simulink model "test2"  (Simulink 7.5)
settings: Solver=ode15s  StartTime=0.0  StopTime=50  RelTol=1e-3
libraries: powerlib x16, powerlib_extras x2
settings Model: Creator=lm  LastModifiedBy=lm

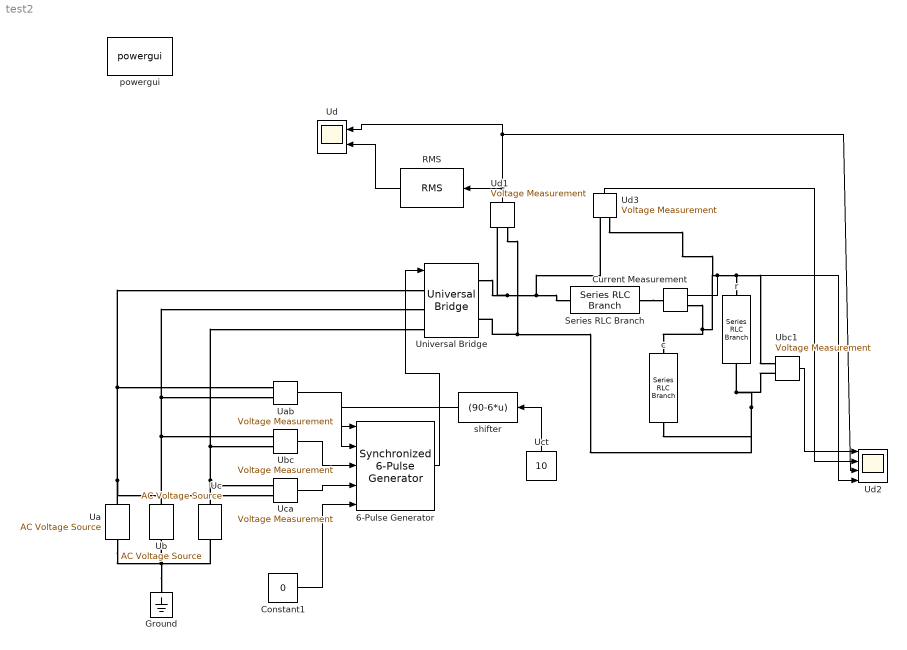
== system test2 ==
  6-Pulse Generator : powerlib_extras/Control  Blocks/Synchronized 6-Pulse Generator  DialogController=POWERSYS.PowerSysDialog  SystemSampleTime=-1  freq=50  pwidth=5  Double_Pulse=on
  Constant1 : Constant  Value=0  OutDataType=fixdt(1, 16)  OutScaling=2^0
  Current Measurement : powerlib/Measurements/Current Measurement  DialogController=POWERSYS.PowerSysDialog  SystemSampleTime=-1  PhasorSimulation=off  OutputType=Complex  PSBequivalent=0
  Ground : powerlib/Elements/Ground  DialogController=POWERSYS.PowerSysDialog  PhysicalDomain=powersysdomain  SubClassName=unknown  LeftPortType=p1  RightPortType=p1  LConnTagsString=a
  RMS : powerlib_extras/Measurements/RMS  DialogController=POWERSYS.PowerSysDialog  SystemSampleTime=-1  f1=60
  Series RLC Branch : powerlib/Elements/Series RLC Branch  DialogController=POWERSYS.PowerSysDialog  PhysicalDomain=powersysdomain  SubClassName=unknown  LeftPortType=p1  RightPortType=p1  LConnTagsString=__new0  RConnTagsString=__new0  BranchType=RL  Resistance=0.2  Inductance=0.2  SetiL0=off  InitialCurrent=0  Capacitance=1e-6  Setx0=off  InitialVoltage=0  Measurements=None
  Ua : powerlib/Electrical Sources/AC Voltage Source  DialogController=POWERSYS.PowerSysDialog  SystemSampleTime=-1  Amplitude=220*sqrt(2)  Phase=0  Frequency=50  SampleTime=0  Measurements=None
  Uab : powerlib/Measurements/Voltage Measurement  DialogController=POWERSYS.PowerSysDialog  SystemSampleTime=-1  PhasorSimulation=off  OutputType=Complex  PSBequivalent=0
  Ub : powerlib/Electrical Sources/AC Voltage Source  DialogController=POWERSYS.PowerSysDialog  SystemSampleTime=-1  Amplitude=220*sqrt(2)  Phase=-120  Frequency=50  SampleTime=0  Measurements=None
  Ubc : powerlib/Measurements/Voltage Measurement  DialogController=POWERSYS.PowerSysDialog  SystemSampleTime=-1  PhasorSimulation=off  OutputType=Complex  PSBequivalent=0
  Ubc1 : powerlib/Measurements/Voltage Measurement  DialogController=POWERSYS.PowerSysDialog  SystemSampleTime=-1  PhasorSimulation=off  OutputType=Complex  PSBequivalent=0
  Uc : powerlib/Electrical Sources/AC Voltage Source  DialogController=POWERSYS.PowerSysDialog  SystemSampleTime=-1  Amplitude=220*sqrt(2)  Phase=-240  Frequency=50  SampleTime=0  Measurements=None
  Uca : powerlib/Measurements/Voltage Measurement  DialogController=POWERSYS.PowerSysDialog  SystemSampleTime=-1  PhasorSimulation=off  OutputType=Complex  PSBequivalent=0
  Uct : Constant  Value=10  OutDataType=fixdt(1, 16)  OutScaling=2^0
  Ud : Scope  NumInputPorts=2
      settings: YMin=-80~1.7e-005  YMax=0~2.125e-005
  Ud1 : powerlib/Measurements/Voltage Measurement  DialogController=POWERSYS.PowerSysDialog  SystemSampleTime=-1  PhasorSimulation=off  OutputType=Complex  PSBequivalent=0
  Ud2 : Scope  NumInputPorts=4
      settings: TimeRange=4  YMin=362~-125~250~361.5  YMax=362.3~175~550~362.6
  Ud3 : powerlib/Measurements/Voltage Measurement  DialogController=POWERSYS.PowerSysDialog  SystemSampleTime=-1  PhasorSimulation=off  OutputType=Complex  PSBequivalent=0
  Universal Bridge : powerlib/Power Electronics/Universal Bridge  DialogController=POWERSYS.PowerSysDialog  SystemSampleTime=-1  Arms=3  SnubberResistance=1e6  SnubberCapacitance=inf  Device=Thyristors  Ron=0.006  Lon=0  ForwardVoltages="[  0  0  ]"  ForwardVoltage=0  GTOparameters=[ 10e-6 , 20e-6 ]  IGBTparameters=[ 1e-6 , 2e-6 ]  Measurements=Device voltages  Measurements_2=None  converterType=Rectifier
  c : powerlib/Elements/Series RLC Branch  DialogController=POWERSYS.PowerSysDialog  PhysicalDomain=powersysdomain  SubClassName=unknown  LeftPortType=p1  RightPortType=p1  LConnTagsString=__new0  RConnTagsString=__new0  BranchType=C  Resistance=1  Inductance=1e-3  SetiL0=off  InitialCurrent=0  Capacitance=0.1  Setx0=off  InitialVoltage=0  Measurements=None
  powergui : powerlib/powergui  Priority=1  SystemSampleTime=-1  SimulationMode=Discrete  SampleTime=50e-6  frequency=60  SPID=off  DisableSnubberDevices=off  DisableRonSwitches=off  DisableVfSwitches=off  SwTol=0  Interpol=off  frequencyindice=0  echomessages=off  HookPort=off  DisplayEquations=off  FunctionMessages=off  EnableUseOfTLC=off  x0status=blocks  RestoreLinks=warning  ResistiveCurrentMeasurement=off  Ylog=off  Xlog=on  ShowGrid=off  save=off  variable=ZData  ZoomFFT=off  StartTime=0.0  cycles=1  DisplayStyle=1  FreqAxis=off  MaxFrequency=1000  frequencyindicesteady=1  display=off  methode=off
  r : powerlib/Elements/Series RLC Branch  DialogController=POWERSYS.PowerSysDialog  PhysicalDomain=powersysdomain  SubClassName=unknown  LeftPortType=p1  RightPortType=p1  LConnTagsString=__new0  RConnTagsString=__new0  BranchType=R  Resistance=1  Inductance=1e-3  SetiL0=off  InitialCurrent=0  Capacitance=1e-6  Setx0=off  InitialVoltage=0  Measurements=None
  shifter : Fcn  Expr=(90-6*u)
  wires:
  Constant1/1 -> 6-Pulse Generator/5
  Uca/1 -> 6-Pulse Generator/4
  Ubc/1 -> 6-Pulse Generator/3
  Uab/1 -> 6-Pulse Generator/2
  Uct/1 -> shifter/1
  shifter/1 -> 6-Pulse Generator/1
  Ud1/1 -> RMS/1, Ud/1, Ud2/3
  RMS/1 -> Ud/2
  6-Pulse Generator/1 -> Universal Bridge/1
  Ubc1/1 -> Ud2/1
  Ud3/1 -> Ud2/2
  Current Measurement/1 -> Ud2/4
  connections:
  Ground/LConn1 -- Ua/LConn1 -- Ub/LConn1 -- Uc/LConn1
  Ua/RConn1 -- Universal Bridge/LConn1 -- Uab/LConn1 -- Uca/LConn2
  Ub/RConn1 -- Universal Bridge/LConn2 -- Uab/LConn2 -- Ubc/LConn1
  Uc/RConn1 -- Universal Bridge/LConn3 -- Ubc/LConn2 -- Uca/LConn1
  Ud3/LConn1 -- Universal Bridge/RConn1 -- Ud1/LConn1 -- Series RLC Branch/LConn1
  Ud1/LConn2 -- Universal Bridge/RConn2 -- Ubc1/LConn2 -- r/LConn1 -- c/RConn1
  Ud3/LConn2 -- r/RConn1 -- Ubc1/LConn1 -- Current Measurement/RConn1 -- c/LConn1
  Series RLC Branch/RConn1 -- Current Measurement/LConn1
